simulink model "lab1SimDom"  (R2023b)
settings: Solver=VariableStepAuto  StartTime=0.0  StopTime=10.0  RelTol=1e-3
values from neighbouring files (symbols this model uses):
  cpp = 1000    [lab1Dom.m]
  Cvs = cps * ros * Vs    (= 9240000)    [lab1Dom.m]
  Cvw = cpp * rop * Vw    (= 150000)    [lab1Dom.m]
  czas_skok = 5000    [lab1Dom.m]
  dFp = 0    [lab1Dom.m]
  dPg = 0    [lab1Dom.m]
  dTzew = 1    [lab1Dom.m]
  Fp0 = FpN * 1.0    (= 0.0694444444444)    [lab1Dom.m]
  Ks = Px/(TsN - TzewN)    (= 133.333333333)    [lab1Dom.m]
  Kw = Px/(TwewN - TsN)    (= 933.333333333)    [lab1Dom.m]
  Pg0 = PgN * 1.0    (= 8000)    [lab1Dom.m]
  rop = 1.2    [lab1Dom.m]
  Ts0 = (Kw*Twew0 + Ks*Tzew0) / (Kw + Ks)    (= 15)    [lab1Dom.m]
  Twew0 = (Pg0 + Tzew0*(cpp*rop*Fp0 + ((Ks*Kw)/(Kw + Ks)))) / (cpp*rop*Fp0 + ((Kw * Ks)/(Kw + Ks)))    (= 20)    [lab1Dom.m]
  Tzew0 = TzewN + 0    (= -20)    [lab1Dom.m]
settings Model: Creator=Michal  LastModifiedBy=Michal
settings DataIOCC: ReturnWorkspaceOutputs=off

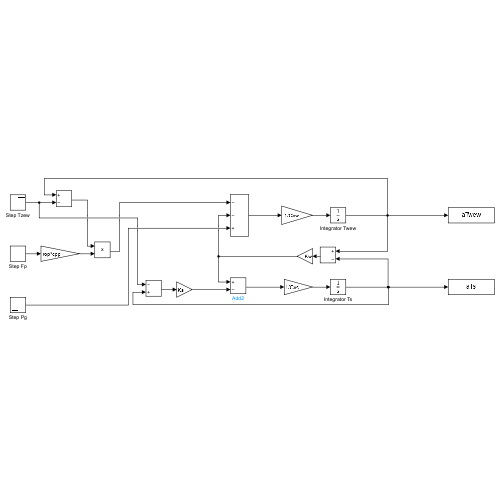
[thumbnail: Simulink's stored preview of the top-level diagram]
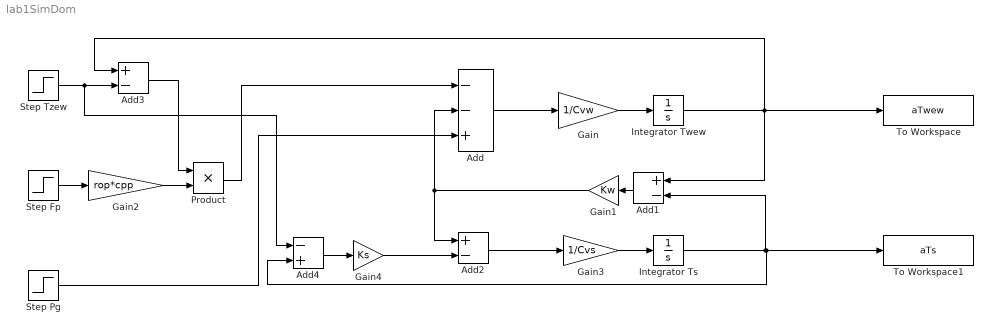
== system lab1SimDom ==
  Add : Sum  Inputs=--+
  Add1 : Sum  Inputs=+-
  Add2 : Sum  Inputs=+-
  Add3 : Sum  Inputs=+-
  Add4 : Sum  Inputs=-+
  Gain : Gain  Gain=1/Cvw
  Gain1 : Gain  Gain=Kw
  Gain2 : Gain  Gain=rop*cpp
  Gain3 : Gain  Gain=1/Cvs
  Gain4 : Gain  Gain=Ks
  Integrator Ts : Integrator  InitialCondition=Ts0
  Integrator Twew : Integrator  InitialCondition=Twew0
  Product : Product
  Step Fp : Step  Time=czas_skok  Before=Fp0  After=Fp0+dFp  SampleTime=0
  Step Pg : Step  Time=czas_skok  Before=Pg0  After=Pg0+dPg  SampleTime=0
  Step Tzew : Step  Time=czas_skok  Before=Tzew0  After=Tzew0+dTzew  SampleTime=0
  To Workspace : ToWorkspace  VariableName=aTwew  SampleTime=-1
  To Workspace1 : ToWorkspace  VariableName=aTs  SampleTime=-1
  wires:
  Integrator Twew/1 -> Add3/1, Add1/1, To Workspace/1
  Gain/1 -> Integrator Twew/1
  Step Pg/1 -> Add/3
  Add/1 -> Gain/1
  Integrator Ts/1 -> Add1/2, Add4/2, To Workspace1/1
  Add1/1 -> Gain1/1
  Gain1/1 -> Add2/1, Add/2
  Add2/1 -> Gain3/1
  Step Fp/1 -> Gain2/1
  Gain2/1 -> Product/2
  Step Tzew/1 -> Add4/1, Add3/2
  Add3/1 -> Product/1
  Product/1 -> Add/1
  Gain3/1 -> Integrator Ts/1
  Add4/1 -> Gain4/1
  Gain4/1 -> Add2/2
